simulink model "A1_FSM"  (R2022a)
settings: Solver=FixedStepAuto  StartTime=0.0  StopTime=inf  FixedStep=0.2  RelTol=1e-3
settings Model: Creator=ArriGE66  LastModifiedBy=jacopo

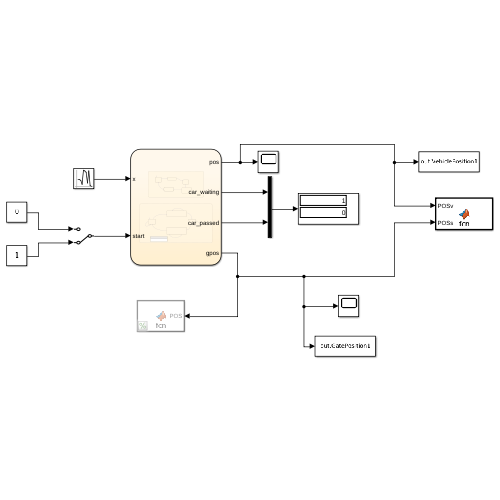
[thumbnail: Simulink's stored preview of the top-level diagram]
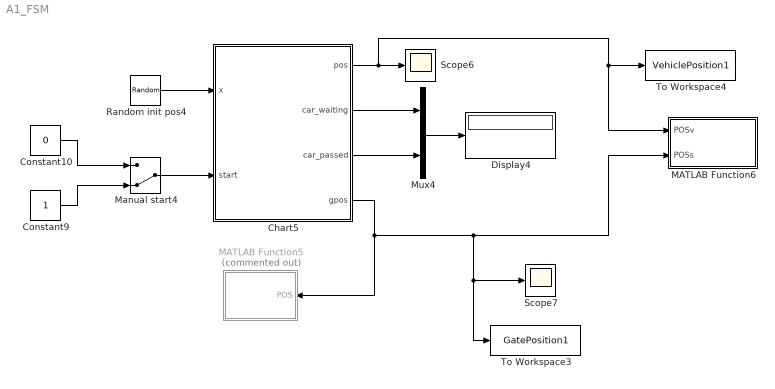
== system A1_FSM ==
  Chart5 : Stateflow chart  TreatAsAtomicUnit=on
  Constant10 : Constant  Value=0
  Constant9 : Constant
  Display4 : Display
  MATLAB Function5 : MATLAB Function  Commented=on  TreatAsAtomicUnit=on
  MATLAB Function6 : MATLAB Function  TreatAsAtomicUnit=on
  Manual start4 : ManualSwitch  CurrentSetting=0
  Mux4 : Mux  Inputs=2
  Random init pos4 : RandomNumber  Mean=-15  Variance=5  SampleTime=0.2
  Scope6 : Scope
  Scope7 : Scope
  To Workspace3 : ToWorkspace  VariableName=GatePosition1  SampleTime=-1
  To Workspace4 : ToWorkspace  VariableName=VehiclePosition1  SampleTime=-1
  wires:
  Chart5/1(pos) -> To Workspace4/1, MATLAB Function6/1(POSv), Scope6/1
  Chart5/4(gpos) -> MATLAB Function5/1(POS), To Workspace3/1, Scope7/1, MATLAB Function6/2(POSs)
  Manual start4/1 -> Chart5/2(start)
  Random init pos4/1 -> Chart5/1(x)
  Constant9/1 -> Manual start4/2
  Constant10/1 -> Manual start4/1
  Mux4/1 -> Display4/1
  Chart5/3(car_passed) -> Mux4/2
  Chart5/2(car_waiting) -> Mux4/1

== matlab function A1_FSM/MATLAB Function5 ==
  data: POS input
function fcn(POS)

    a = 0.5;
    c = 2;
    L = 4;
    b = a + L*cos(POS);
    d = c + L*sin(POS);
    clf
    plot([a b], [c d], 'r', 'LineWidth', 2)
    hold on
    plot([0.5 0.5], [0 2], 'b', 'LineWidth', 8)
    xlim([0 6])
    ylim([0 6])
    
end

== matlab function A1_FSM/MATLAB Function6 ==
  data: POSv input; POSs input
function fcn(POSv, POSs)

    a = 0;
    c = 2;
    L = 4;
    b = a + L*cos(POSs);
    d = c + L*sin(POSs);
    clf
    plot3([0 0], [a b], [c d], 'r', 'LineWidth', 2)
    hold on
    plot3([0 0], [0 0], [0 2], 'b', 'LineWidth', 8)
    hold on
    plot3(POSv, 2, 0, '*k', 'LineWidth', 10)
    grid on
    xlim([-6 1])
    ylim([-0.5 6])
    zlim([0 6])
    
end

== stateflow chart A1_FSM/Chart5 ==
  state superstate1 [parallel]
    settings: executionOrder=1
    state idle
      init = x;
      pos = init;
      car_waiting = 0;
      car_passed = 0;
    state approaching
      pos = init + v*elapsed(sec);
    state stop
      tmp = pos;
      car_waiting = 1;
      car_passed = 0;
    state pass
      pos = tmp+v*elapsed(sec);
      car_waiting = 0;
      ex:
      pos = tmp + v*elapsed(sec);
      tmp = pos;
    state passed
      pos = tmp + v*elapsed(sec);
      car_passed = 1;
    (default) -> idle
    approaching -> stop : [pos >= 0]
    idle -> approaching : [start == 1]
    passed -> idle : [after(10, sec)]
    stop -> pass : [gate_up == 1]
    pass -> passed : [pos >= gate_end]
  state superstate2 [parallel]
    settings: executionOrder=2
    state raising
      [gpos, gate_up, Tc] = gateAction(T, raise, gpos, Tc, 0);
    state up
      oldpos = gpos;
      Tc = 0;
    state down
      gpos = 0;
      gate_up = 0;
      raise = 0;
      Tc = 0;
    state lowering
      [gpos, gate_up, Tc] = gateAction(T, raise, gpos, Tc, oldpos);
    raising -> raising [order 1] : [gate_up == 0 || gate_up > 1] {raise = 1, T = elapsed(sec)}
    raising -> up [order 2] : [gate_up == 1]
    down -> raising [order 2] : [car_waiting == 1] {raise = 1, T = elapsed(sec)}
    (default) -> down
    up -> up [order 1] : [car_passed == 0]
    down -> down [order 1] : [car_waiting == 0]
    lowering -> down [order 2] : [gate_up == 0]
    up -> lowering [order 2] : [car_passed == 1] {raise = -1, T = elapsed(sec)}
    lowering -> lowering [order 1] : [gate_up > 1] {raise = -1, T = elapsed(sec)}
  data: vpos function_output double; vgu function_output; vt function_input; vr function_input; vposin function_input; Tcum function_input; t function_output; oldpos function_input; gate_end local =3; v local double =1; pos output; car_waiting output; car_passed output; init local; x input; start input; tmp local; gpos output; T local; raise local; gate_up local; Tc local; oldpos local
  function [vpos, vgu, t] = gateAction(vt, vr, vposin, Tcum, oldpos):
    | function [vpos, vgu, t] = gateAction(vt, vr, vposin, Tcum, oldpos)
    | 
    | % vt is time
    | % vr is raise command
    | 
    | % vpos is pos
    | % vgu is gate_up
    | 
    | % gate specs
    | wmax = 4*pi/180;                                                            % rad/s, maximum angular velocity of gate
    | dwmax = 1*pi/180;                                                           % rad/s, maximum angular acceleration of gate
    | DC = 0;                                                                     % rad,   down condition
    | UC = pi/2;                                                                  % rad,   up condition
    | 
    | 
    | t = Tcum + vt;
    | 
    | if vr == 1
    |     vpos = 1/2*dwmax*t^2;
    | 
    | elseif vr == - 1
    |     vpos = oldpos - 1/2*dwmax*t^2;
    | 
    | else
    |     vpos = vposin;
    | end
    | 
    | if abs(vpos - DC) < 1e-2
    |     vgu = 0;
    | elseif abs(vpos - UC) < 1e-2
    |     vgu = 1;
    | else
    |     vgu = 2;
    | end
    | 
    | 
    | end
